simulink model "SingleTrackCANoe"  (R2021b)
settings: Solver=ode1  StartTime=0  StopTime=2  FixedStep=1.0000000000000000e-003  RelTol=1e-3
InitFcn:
  | sampleTime = str2double(get_param(bdroot, 'FixedStep'));
undefined symbols (not defined in the file or in its folder): AccPedalPos, BrakePedalPos, BrakeSwitch, DiscIntNeverNeededParam, DYNA4, EngSpd, IgnitionSwitch, InitialGear, InitialSpeed, IntendedEngTrq, LeftIndicator, MainBrakePress, MaxGear, MDL, MinGear, RefAcc, RefLane, RefLatPos, RefPath, RefPathCurv, RefSpd, RefSpdPreview, RefSpdRetrospect, RightIndicator, SteeringWheelAng, SteeringWheelTrq, UserDefinedRefValue, vm_const
libraries: UtilitiesLibrary x62, simulink x18, WheelSystemModules x14, LongitudinalControllerModules x13, LateralControllerModules x7, AnimationBusselectorModules x5, EnvironmentModules x5, BasicEngineControlModules x5, MiscellaneousControlModules x5, Animation3Modules x4, AuxiliariesModules x4, ReducedTireModules x4
(part 29 of 34)

== system SingleTrackCANoe/SimulationModel/Vehicle/Drivetrain/DrivetrainPhysics/DrivetrainPhysicsOutputs/RearLeftShaftOutput ==
  In1 : Inport
  Bus Selector : BusSelector  OutputSignals=Trq,RotSpd,RotAcc[rad/s**2],DTrqRotAng,DTrqRotSpd,Inrt[kg*m**2],FrictionTrq[Nm]
  RearLeftShaftOutput : Subsystem  Tag=TESIS DYNAware Interface Block  mask{NeedsUpdate=off, SignalInfo=|}
      mask SignalInfo=|
      | {
      |   "Version": "4.6",
      |   "MuxedOutputBusName": "RearLeftShaft",
      |   "MuxedInputBusName": "input",
      |   "MuxedInputSelected": false,
      |   "MuxedOutputSelected": true,
      |   "SignalData": [
      |     {
      |       "initialValue": "0.0",
      |       "name": "Trq[Nm]",
      |       "comment": "",
      |       "minString": "",
      |       "maxString": "",
      |       "width": 1,
      |       "dataType": 0,
      |       "signalType": 0,
      |       "createSignal": false,
      |       "outputName": "Trq[Nm]",
      |       "generateSignalAccessBlock": false,
      |       "accessId": "$(parentId).$(blockName).$(outputName)"
      |     },
      |     {
      |       "initialValue": "0.0",
      |       "name": "RotSpdDifferentialOut[rad/s]",
      |       "comment": "",
      |       "minString": "",
      |       "maxString": "",
      |       "width": 1,
      |       "dataType": 0,
      |       "signalType": 0,
      |       "createSignal": false,
      |       "outputName": "RotSpdDifferentialOut[rad/s]",
      |       "generateSignalAccessBlock": false,
      |       "accessId": "$(parentId).$(blockName).$(outputName)"
      |     },
      |     {
      |       "initialValue": "0.0",
      |       "name": "RotAcc[rad/s**2]",
      |       "comment": "",
      |       "minString": "",
      |       "maxString": "",
      |       "width": 1,
      |       "dataType": 0,
      |       "signalType": 0,
      |       "createSignal": false,
      |       "outputName": "RotAcc[rad/s**2]",
      |       "generateSignalAccessBlock": false,
      |       "accessId": "$(parentId).$(blockName).$(outputName)"
      |     },
      |     {
      |       "initialValue": "0.0",
      |       "name": "DerivativeOfTrq_wrt_RotAng[Nm/rad]",
      |       "comment": "",
      |       "minString": "",
      |       "maxString": "",
      |       "width": 1,
      |       "dataType": 0,
      |       "signalType": 0,
      |       "createSignal": false,
      |       "outputName": "DerivativeOfTrq_wrt_RotAng[Nm/rad]",
      |       "generateSignalAccessBlock": false,
      |       "accessId": "$(parentId).$(blockName).$(outputName)"
      |     },
      |     {
      |       "initialValue": "0.0",
      |       "name": "DerivativeOfTrq_wrt_WheelSpd[Nm/(rad/s)]",
      |       "comment": "",
      |       "minString": "",
      |       "maxString": "",
      |       "width": 1,
      |       "dataType": 0,
      |       "signalType": 0,
      |       "createSignal": false,
      |       "outputName": "DerivativeOfTrq_wrt_WheelSpd[Nm/(rad/s)]",
      |       "generateSignalAccessBlock": false,
      |       "accessId": "$(parentId).$(blockName).$(outputName)"
      |     },
      |     {
      |       "initialValue": "0.0",
      |       "name": "AddInrt[kg*m**2]",
      |       "comment": "",
      |       "minString": "",
      |       "maxString": "",
      |       "width": 1,
      |       "dataType": 0,
      |       "signalType": 0,
      |       "createSignal": false,
      |       "outputName": "AddInrt[kg*m**2]",
      |       "generateSignalAccessBlock": false,
      |       "accessId": "$(parentId).$(blockName).$(outputName)"
      |     },
      |     {
      |       "initialValue": "0.0",
      |       "name": "FrictionTrq[Nm]",
      |       "comment": "",
      |       "minString": "",
      |       "maxString": "",
      |       "width": 1,
      |       "dataType": 0,
      |       "signalType": 0,
      |       "createSignal": false,
      |       "outputName": "FrictionTrq[Nm]",
      |       "generateSignalAccessBlock": false,
      |       "accessId": "$(parentId).$(blockName).$(outputName)"
      |     }
      |   ]
      | }
      mask prompts: NeedsUpdate "Specify, if subsystem content needs to be updated"; SignalInfo "Signal Info (json)"
      mask help: DYNA4 Interface Block Version 4.6
      mask init:
      | blockName = get_param(gcbh, 'Name');
      | parentId = DYNA4.ModelHandling.AccessID.getFromHierarchy(gcbh);
      | TD.InterfaceBlock.ModelCallbacks.GenerateContent(gcb);
      settings: DeleteFcn=TD.InterfaceBlock.ModelCallbacks.CloseGUI( gcbh );  NameChangeFcn=TD.InterfaceBlock.ModelCallbacks.BlockRenamedHandler(gcbh);  OpenFcn=TD.InterfaceBlock.ModelCallbacks.OpenGUI( gcbh );  CloseFcn=TD.InterfaceBlock.ModelCallbacks.CloseGUI( gcbh );
      mask Display:
      | image('InterfaceBlock.png','center');
      | port_label('input',1, 'Trq[Nm]');
      | port_label('input',2, 'RotSpdDifferentialOut[rad/s]');
      | port_label('input',3, 'RotAcc[rad/s**2]');
      | port_label('input',4, 'DerivativeOfTrq_wrt_RotAng[Nm/rad]');
      | port_label('input',5, 'DerivativeOfTrq_wrt_WheelSpd[Nm/(rad/s)]');
      | port_label('input',6, 'AddInrt[kg*m**2]');
      | port_label('input',7, 'FrictionTrq[Nm]');
      | port_label('output',1, 'RearLeftShaft');
  RearLeftShaft : Outport  VectorParamsAs1DForOutWhenUnconnected=off
  wires:
  RearLeftShaftOutput/1(RearLeftShaft___UNIQUE_1) -> RearLeftShaft/1
  In1/1 -> Bus Selector/1
  Bus Selector/1 -> RearLeftShaftOutput/1(Trq[Nm]___UNIQUE_1)  "<Trq>"
  Bus Selector/7 -> RearLeftShaftOutput/7(FrictionTrq[Nm]___UNIQUE_1)  "<FrictionTrq[Nm]>"
  Bus Selector/6 -> RearLeftShaftOutput/6(AddInrt[kg*m**2]___UNIQUE_1)  "<Inrt[kg*m**2]>"
  Bus Selector/4 -> RearLeftShaftOutput/4(DerivativeOfTrq_wrt_RotAng[Nm/rad]___UNIQUE_1)  "<DTrqRotAng>"
  Bus Selector/5 -> RearLeftShaftOutput/5(DerivativeOfTrq_wrt_WheelSpd[Nm/(rad/s)]___UNIQUE_1)  "<DTrqRotSpd>"
  Bus Selector/3 -> RearLeftShaftOutput/3(RotAcc[rad/s**2]___UNIQUE_1)  "<RotAcc[rad/s**2]>"
  Bus Selector/2 -> RearLeftShaftOutput/2(RotSpdDifferentialOut[rad/s]___UNIQUE_1)  "<RotSpd>"

== system SingleTrackCANoe/SimulationModel/Vehicle/Drivetrain/DrivetrainPhysics/DrivetrainPhysicsOutputs/RearRightShaftOutput ==
  In1 : Inport
  Bus Selector : BusSelector  OutputSignals=Trq,RotSpd,RotAcc[rad/s**2],DTrqRotAng,DTrqRotSpd,Inrt[kg*m**2],FrictionTrq[Nm]
  RearRightShaftOutput : Subsystem  Tag=TESIS DYNAware Interface Block  mask{NeedsUpdate=off, SignalInfo=|}
      mask SignalInfo=|
      | {
      |   "Version": "4.6",
      |   "MuxedOutputBusName": "RearRightShaft",
      |   "MuxedInputBusName": "input",
      |   "MuxedInputSelected": false,
      |   "MuxedOutputSelected": true,
      |   "SignalData": [
      |     {
      |       "initialValue": "0.0",
      |       "name": "Trq[Nm]",
      |       "comment": "",
      |       "minString": "",
      |       "maxString": "",
      |       "width": 1,
      |       "dataType": 0,
      |       "signalType": 0,
      |       "createSignal": false,
      |       "outputName": "Trq[Nm]",
      |       "generateSignalAccessBlock": false,
      |       "accessId": "$(parentId).$(blockName).$(outputName)"
      |     },
      |     {
      |       "initialValue": "0.0",
      |       "name": "RotSpdDifferentialOut[rad/s]",
      |       "comment": "",
      |       "minString": "",
      |       "maxString": "",
      |       "width": 1,
      |       "dataType": 0,
      |       "signalType": 0,
      |       "createSignal": false,
      |       "outputName": "RotSpdDifferentialOut[rad/s]",
      |       "generateSignalAccessBlock": false,
      |       "accessId": "$(parentId).$(blockName).$(outputName)"
      |     },
      |     {
      |       "initialValue": "0.0",
      |       "name": "RotAcc[rad/s**2]",
      |       "comment": "",
      |       "minString": "",
      |       "maxString": "",
      |       "width": 1,
      |       "dataType": 0,
      |       "signalType": 0,
      |       "createSignal": false,
      |       "outputName": "RotAcc[rad/s**2]",
      |       "generateSignalAccessBlock": false,
      |       "accessId": "$(parentId).$(blockName).$(outputName)"
      |     },
      |     {
      |       "initialValue": "0.0",
      |       "name": "DerivativeOfTrq_wrt_RotAng[Nm/rad]",
      |       "comment": "",
      |       "minString": "",
      |       "maxString": "",
      |       "width": 1,
      |       "dataType": 0,
      |       "signalType": 0,
      |       "createSignal": false,
      |       "outputName": "DerivativeOfTrq_wrt_RotAng[Nm/rad]",
      |       "generateSignalAccessBlock": false,
      |       "accessId": "$(parentId).$(blockName).$(outputName)"
      |     },
      |     {
      |       "initialValue": "0.0",
      |       "name": "DerivativeOfTrq_wrt_WheelSpd[Nm/(rad/s)]",
      |       "comment": "",
      |       "minString": "",
      |       "maxString": "",
      |       "width": 1,
      |       "dataType": 0,
      |       "signalType": 0,
      |       "createSignal": false,
      |       "outputName": "DerivativeOfTrq_wrt_WheelSpd[Nm/(rad/s)]",
      |       "generateSignalAccessBlock": false,
      |       "accessId": "$(parentId).$(blockName).$(outputName)"
      |     },
      |     {
      |       "initialValue": "0.0",
      |       "name": "AddInrt[kg*m**2]",
      |       "comment": "",
      |       "minString": "",
      |       "maxString": "",
      |       "width": 1,
      |       "dataType": 0,
      |       "signalType": 0,
      |       "createSignal": false,
      |       "outputName": "AddInrt[kg*m**2]",
      |       "generateSignalAccessBlock": false,
      |       "accessId": "$(parentId).$(blockName).$(outputName)"
      |     },
      |     {
      |       "initialValue": "0.0",
      |       "name": "FrictionTrq[Nm]",
      |       "comment": "",
      |       "minString": "",
      |       "maxString": "",
      |       "width": 1,
      |       "dataType": 0,
      |       "signalType": 0,
      |       "createSignal": false,
      |       "outputName": "FrictionTrq[Nm]",
      |       "generateSignalAccessBlock": false,
      |       "accessId": "$(parentId).$(blockName).$(outputName)"
      |     }
      |   ]
      | }
      mask prompts: NeedsUpdate "Specify, if subsystem content needs to be updated"; SignalInfo "Signal Info (json)"
      mask help: DYNA4 Interface Block Version 4.6
      mask init:
      | blockName = get_param(gcbh, 'Name');
      | parentId = DYNA4.ModelHandling.AccessID.getFromHierarchy(gcbh);
      | TD.InterfaceBlock.ModelCallbacks.GenerateContent(gcb);
      settings: DeleteFcn=TD.InterfaceBlock.ModelCallbacks.CloseGUI( gcbh );  NameChangeFcn=TD.InterfaceBlock.ModelCallbacks.BlockRenamedHandler(gcbh);  OpenFcn=TD.InterfaceBlock.ModelCallbacks.OpenGUI( gcbh );  CloseFcn=TD.InterfaceBlock.ModelCallbacks.CloseGUI( gcbh );
      mask Display:
      | image('InterfaceBlock.png','center');
      | port_label('input',1, 'Trq[Nm]');
      | port_label('input',2, 'RotSpdDifferentialOut[rad/s]');
      | port_label('input',3, 'RotAcc[rad/s**2]');
      | port_label('input',4, 'DerivativeOfTrq_wrt_RotAng[Nm/rad]');
      | port_label('input',5, 'DerivativeOfTrq_wrt_WheelSpd[Nm/(rad/s)]');
      | port_label('input',6, 'AddInrt[kg*m**2]');
      | port_label('input',7, 'FrictionTrq[Nm]');
      | port_label('output',1, 'RearRightShaft');
  RearRightShaft : Outport  VectorParamsAs1DForOutWhenUnconnected=off
  wires:
  RearRightShaftOutput/1(RearRightShaft___UNIQUE_1) -> RearRightShaft/1
  In1/1 -> Bus Selector/1
  Bus Selector/1 -> RearRightShaftOutput/1(Trq[Nm]___UNIQUE_1)  "<Trq>"
  Bus Selector/7 -> RearRightShaftOutput/7(FrictionTrq[Nm]___UNIQUE_1)  "<FrictionTrq[Nm]>"
  Bus Selector/6 -> RearRightShaftOutput/6(AddInrt[kg*m**2]___UNIQUE_1)  "<Inrt[kg*m**2]>"
  Bus Selector/4 -> RearRightShaftOutput/4(DerivativeOfTrq_wrt_RotAng[Nm/rad]___UNIQUE_1)  "<DTrqRotAng>"
  Bus Selector/5 -> RearRightShaftOutput/5(DerivativeOfTrq_wrt_WheelSpd[Nm/(rad/s)]___UNIQUE_1)  "<DTrqRotSpd>"
  Bus Selector/3 -> RearRightShaftOutput/3(RotAcc[rad/s**2]___UNIQUE_1)  "<RotAcc[rad/s**2]>"
  Bus Selector/2 -> RearRightShaftOutput/2(RotSpdDifferentialOut[rad/s]___UNIQUE_1)  "<RotSpd>"

== system SingleTrackCANoe/SimulationModel/Vehicle/Drivetrain/DrivetrainPhysics/DrivetrainPhysicsOutputs/TotalRatio ==
  TransmissionStates : Inport
  OutputDriveRatio : Inport  Port=2
  Bus Selector16 : BusSelector  OutputSignals=Ratio[-]
  Product : Product  RndMeth=Zero
  TotalRatio : Outport  VectorParamsAs1DForOutWhenUnconnected=off
  wires:
  Product/1 -> TotalRatio/1
  OutputDriveRatio/1 -> Product/2
  TransmissionStates/1 -> Bus Selector16/1
  Bus Selector16/1 -> Product/1  "<Ratio[-]>"

== system SingleTrackCANoe/SimulationModel/Vehicle/Drivetrain/DrivetrainPhysics/DrivetrainPhysicsOutputs/TransferCaseOutput ==
  TransferCaseStates : Inport
  Bus Selector : BusSelector  OutputSignals=TrqDistributionFac[0_1]
  TransferCaseOutput : Subsystem  Tag=TESIS DYNAware Interface Block  mask{NeedsUpdate=off, SignalInfo=|}
      mask SignalInfo=|
      | {
      |   "Version": "4.6",
      |   "MuxedOutputBusName": "TransferCase",
      |   "MuxedInputBusName": "input",
      |   "MuxedInputSelected": false,
      |   "MuxedOutputSelected": true,
      |   "SignalData": {
      |     "initialValue": "0.0",
      |     "name": "TrqDistributionFac[0_1]",
      |     "comment": "",
      |     "minString": "",
      |     "maxString": "",
      |     "width": 1,
      |     "dataType": 0,
      |     "signalType": 0,
      |     "createSignal": false,
      |     "outputName": "TrqDistributionFac[0_1]",
      |     "generateSignalAccessBlock": false,
      |     "accessId": "$(parentId).$(blockName).$(outputName)"
      |   }
      | }
      mask prompts: NeedsUpdate "Specify, if subsystem content needs to be updated"; SignalInfo "Signal Info (json)"
      mask help: DYNA4 Interface Block Version 4.6
      mask init:
      | blockName = get_param(gcbh, 'Name');
      | parentId = DYNA4.ModelHandling.AccessID.getFromHierarchy(gcbh);
      | TD.InterfaceBlock.ModelCallbacks.GenerateContent(gcb);
      settings: DeleteFcn=TD.InterfaceBlock.ModelCallbacks.CloseGUI( gcbh );  NameChangeFcn=TD.InterfaceBlock.ModelCallbacks.BlockRenamedHandler(gcbh);  OpenFcn=TD.InterfaceBlock.ModelCallbacks.OpenGUI( gcbh );  CloseFcn=TD.InterfaceBlock.ModelCallbacks.CloseGUI( gcbh );
      mask Display:
      | image('InterfaceBlock.png','center');
      | port_label('input',1, 'TrqDistributionFac[0_1]');
      | port_label('output',1, 'TransferCase');
  TransferCase : Outport  VectorParamsAs1DForOutWhenUnconnected=off
  wires:
  TransferCaseStates/1 -> Bus Selector/1
  TransferCaseOutput/1(TransferCase___UNIQUE_1) -> TransferCase/1
  Bus Selector/1 -> TransferCaseOutput/1(TrqDistributionFac[0_1]___UNIQUE_1)  "<TrqDistributionFac[0_1]>"

== system SingleTrackCANoe/SimulationModel/Vehicle/Drivetrain/DrivetrainPhysics/DrivetrainPhysicsOutputs/TransmissionOutput ==
  TransmissionStates : Inport
  Bus Selector : BusSelector  OutputSignals=NumFwdGears,Type[-],Gear[-4;20],InSpd[rad/s],OutSpd[rad/s],GearChangeTimeConst
  TransmissionOutput : Subsystem  Tag=TESIS DYNAware Interface Block  mask{NeedsUpdate=off, SignalInfo=|}
      mask SignalInfo=|
      | {
      |   "Version": "4.6",
      |   "MuxedOutputBusName": "Transmission",
      |   "MuxedInputBusName": "input",
      |   "MuxedInputSelected": false,
      |   "MuxedOutputSelected": true,
      |   "SignalData": [
      |     {
      |       "initialValue": "0.0",
      |       "name": "NumFwdGears[-]",
      |       "comment": "",
      |       "minString": "",
      |       "maxString": "",
      |       "width": 1,
      |       "dataType": 0,
      |       "signalType": 0,
      |       "createSignal": false,
      |       "outputName": "NumFwdGears[-]",
      |       "generateSignalAccessBlock": false,
      |       "accessId": "$(parentId).$(blockName).$(outputName)"
      |     },
      |     {
      |       "initialValue": "0.0",
      |       "name": "Type[-]",
      |       "comment": "",
      |       "minString": "",
      |       "maxString": "",
      |       "width": 1,
      |       "dataType": 0,
      |       "signalType": 0,
      |       "createSignal": false,
      |       "outputName": "Type[-]",
      |       "generateSignalAccessBlock": false,
      |       "accessId": "$(parentId).$(blockName).$(outputName)"
      |     },
      |     {
      |       "initialValue": "0.0",
      |       "name": "Gear[-4;20]",
      |       "comment": "",
      |       "minString": "",
      |       "maxString": "",
      |       "width": 1,
      |       "dataType": 0,
      |       "signalType": 0,
      |       "createSignal": false,
      |       "outputName": "Gear[-4;20]",
      |       "generateSignalAccessBlock": false,
      |       "accessId": "$(parentId).$(blockName).$(outputName)"
      |     },
      |     {
      |       "initialValue": "0.0",
      |       "name": "InSpd[rad/s]",
      |       "comment": "",
      |       "minString": "",
      |       "maxString": "",
      |       "width": 1,
      |       "dataType": 0,
      |       "signalType": 0,
      |       "createSignal": false,
      |       "outputName": "InSpd[rad/s]",
      |       "generateSignalAccessBlock": false,
      |       "accessId": "$(parentId).$(blockName).$(outputName)"
      |     },
      |     {
      |       "initialValue": "0.0",
      |       "name": "OutSpd[rad/s]",
      |       "comment": "",
      |       "minString": "",
      |       "maxString": "",
      |       "width": 1,
      |       "dataType": 0,
      |       "signalType": 0,
      |       "createSignal": false,
      |       "outputName": "OutSpd[rad/s]",
      |       "generateSignalAccessBlock": false,
      |       "accessId": "$(parentId).$(blockName).$(outputName)"
      |     },
      |     {
      |       "initialValue": "0.0",
      |       "name": "GearChangeTimeConst[s]",
      |       "comment": "",
      |       "minString": "",
      |       "maxString": "",
      |       "width": 1,
      |       "dataType": 0,
      |       "signalType": 0,
      |       "createSignal": false,
      |       "outputName": "GearChangeTimeConst[s]",
      |       "generateSignalAccessBlock": false,
      |       "accessId": "$(parentId).$(blockName).$(outputName)"
      |     }
      |   ]
      | }
      mask prompts: NeedsUpdate "Specify, if subsystem content needs to be updated"; SignalInfo "Signal Info (json)"
      mask help: DYNA4 Interface Block Version 4.6
      mask init:
      | blockName = get_param(gcbh, 'Name');
      | parentId = DYNA4.ModelHandling.AccessID.getFromHierarchy(gcbh);
      | TD.InterfaceBlock.ModelCallbacks.GenerateContent(gcb);
      settings: DeleteFcn=TD.InterfaceBlock.ModelCallbacks.CloseGUI( gcbh );  NameChangeFcn=TD.InterfaceBlock.ModelCallbacks.BlockRenamedHandler(gcbh);  OpenFcn=TD.InterfaceBlock.ModelCallbacks.OpenGUI( gcbh );  CloseFcn=TD.InterfaceBlock.ModelCallbacks.CloseGUI( gcbh );
      mask Display:
      | image('InterfaceBlock.png','center');
      | port_label('input',1, 'NumFwdGears[-]');
      | port_label('input',2, 'Type[-]');
      | port_label('input',3, 'Gear[-4;20]');
      | port_label('input',4, 'InSpd[rad/s]');
      | port_label('input',5, 'OutSpd[rad/s]');
      | port_label('input',6, 'GearChangeTimeConst[s]');
      | port_label('output',1, 'Transmission');
  Transmission : Outport  VectorParamsAs1DForOutWhenUnconnected=off
  wires:
  TransmissionOutput/1(Transmission___UNIQUE_1) -> Transmission/1
  TransmissionStates/1 -> Bus Selector/1
  Bus Selector/2 -> TransmissionOutput/2(Type[-]___UNIQUE_1)  "<Type[-]>"
  Bus Selector/1 -> TransmissionOutput/1(NumFwdGears[-]___UNIQUE_1)  "<NumFwdGears>"
  Bus Selector/6 -> TransmissionOutput/6(GearChangeTimeConst[s]___UNIQUE_1)  "<GearChangeTimeConst>"
  Bus Selector/3 -> TransmissionOutput/3(Gear[-4;20]___UNIQUE_1)  "<Gear[-4;20]>"
  Bus Selector/4 -> TransmissionOutput/4(InSpd[rad/s]___UNIQUE_1)  "<InSpd[rad/s]>"
  Bus Selector/5 -> TransmissionOutput/5(OutSpd[rad/s]___UNIQUE_1)  "<OutSpd[rad/s]>"

== system SingleTrackCANoe/SimulationModel/Vehicle/WheelSystem/FrontLeftWheelSystem/Tire/DynaComponentInfo ==

== system SingleTrackCANoe/SimulationModel/Vehicle/WheelSystem/FrontLeftWheelSystem/Tire/InputFromCTRL ==
  fromCTRL : Inport
  TDBusSelector : BusSelector  OutputSignals=AddRoadElev[m],RoadFrictionScaling[0_2],AddLongRoadSlope[-],AddLatRoadSlope[-],LocalRoadSysSwitch[0;1]
  __TDD__AddLatRoadSlope[-] : Demux  Outputs=[1]
  __TDD__AddLongRoadSlope[-] : Demux  Outputs=[1]
  __TDD__AddRoadElev[m] : Demux  Outputs=[1]
  __TDD__LocalRoadSysSwitch[0;1] : Demux  Outputs=[1]
  __TDD__RoadFrictionScaling[0_2] : Demux  Outputs=[1]
  AddRoadElev[m]___UNIQUE_1 : Outport  Description=|  PortDimensions=[1]  VectorParamsAs1DForOutWhenUnconnected=off
      | <name>AddRoadElev[m]</name>
      | <comment></comment>
  RoadFrictionScaling[0_2]___UNIQUE_1 : Outport  Description=|  Port=2  PortDimensions=[1]  VectorParamsAs1DForOutWhenUnconnected=off
      | <name>RoadFrictionScaling[0_2]</name>
      | <comment></comment>
  AddLongRoadSlope[-]___UNIQUE_1 : Outport  Description=|  Port=3  PortDimensions=[1]  VectorParamsAs1DForOutWhenUnconnected=off
      | <name>AddLongRoadSlope[-]</name>
      | <comment></comment>
  AddLatRoadSlope[-]___UNIQUE_1 : Outport  Description=|  Port=4  PortDimensions=[1]  VectorParamsAs1DForOutWhenUnconnected=off
      | <name>AddLatRoadSlope[-]</name>
      | <comment></comment>
  LocalRoadSysSwitch[0;1]___UNIQUE_1 : Outport  Description=|  Port=5  PortDimensions=[1]  VectorParamsAs1DForOutWhenUnconnected=off
      | <name>LocalRoadSysSwitch[0;1]</name>
      | <comment></comment>
  wires:
  fromCTRL/1 -> TDBusSelector/1
  TDBusSelector/1 -> __TDD__AddRoadElev[m]/1  "<AddRoadElev[m]>"
  TDBusSelector/2 -> __TDD__RoadFrictionScaling[0_2]/1  "<RoadFrictionScaling[0_2]>"
  TDBusSelector/3 -> __TDD__AddLongRoadSlope[-]/1  "<AddLongRoadSlope[-]>"
  TDBusSelector/4 -> __TDD__AddLatRoadSlope[-]/1  "<AddLatRoadSlope[-]>"
  TDBusSelector/5 -> __TDD__LocalRoadSysSwitch[0;1]/1  "<LocalRoadSysSwitch[0;1]>"
  __TDD__AddRoadElev[m]/1 -> AddRoadElev[m]___UNIQUE_1/1  "AddRoadElev[m]"
  __TDD__RoadFrictionScaling[0_2]/1 -> RoadFrictionScaling[0_2]___UNIQUE_1/1  "RoadFrictionScaling[0_2]"
  __TDD__AddLongRoadSlope[-]/1 -> AddLongRoadSlope[-]___UNIQUE_1/1  "AddLongRoadSlope[-]"
  __TDD__AddLatRoadSlope[-]/1 -> AddLatRoadSlope[-]___UNIQUE_1/1  "AddLatRoadSlope[-]"
  __TDD__LocalRoadSysSwitch[0;1]/1 -> LocalRoadSysSwitch[0;1]___UNIQUE_1/1  "LocalRoadSysSwitch[0;1]"

== system SingleTrackCANoe/SimulationModel/Vehicle/WheelSystem/FrontLeftWheelSystem/Tire/InputFromChassis ==
  fromChassis : Inport
  TDBusSelector : BusSelector  OutputSignals=VehicleBody.PosAxleSys(WorldSys),VehicleBody.RotMatrix(WorldSys)[-],WheelSystem.WheelRotAxis(VehSys)[-],WheelSystem.TirePos(AxleSys)[m],WheelSystem.TireVel_wrt_WorldSys(VehSys)[m/s],WheelSystem.WheelRotVel_wrt_WorldSys(VehSys)[rad/s],VehicleBody.Vel_wrt_WorldSys(VehSys)[m/s],WheelSystem.WheelRotMatrix(WorldSys)[-],WheelSystem.TireDefl[m]
  __TDD__PosAxleSys(WorldSys) : Demux  Outputs=1
  __TDD__RotMatrix(WorldSys)[-] : Demux  Outputs=[9]
  __TDD__TireDefl[m] : Demux  Outputs=[1]
  __TDD__TirePos(AxleSys)[m] : Demux  Outputs=1
  __TDD__TireVel_wrt_WorldSys(VehSys)[m/s] : Demux  Outputs=[3]
  __TDD__Vel_wrt_WorldSys(VehSys)[m/s] : Demux  Outputs=[3]
  __TDD__WheelRotAxis(VehSys)[-] : Demux  Outputs=[3]
  __TDD__WheelRotMatrix(WorldSys)[-] : Demux  Outputs=[9]
  __TDD__WheelRotVel_wrt_WorldSys(VehSys)[rad/s] : Demux  Outputs=[3]
  PosAxleSys(WorldSys)___UNIQUE_1 : Outport  Description=|  VectorParamsAs1DForOutWhenUnconnected=off
      | <name>VehicleBody.PosAxleSys(WorldSys)</name>
      | <comment></comment>
  RotMatrix(WorldSys)[-]___UNIQUE_1 : Outport  Description=|  Port=2  PortDimensions=[9]  VectorParamsAs1DForOutWhenUnconnected=off
      | <name>VehicleBody.RotMatrix(WorldSys)[-]</name>
      | <comment></comment>
  WheelRotAxis(VehSys)[-]___UNIQUE_1 : Outport  Description=|  Port=3  PortDimensions=[3]  VectorParamsAs1DForOutWhenUnconnected=off
      | <name>WheelSystem.WheelRotAxis(VehSys)[-]</name>
      | <comment></comment>
  TirePos(AxleSys)[m]___UNIQUE_1 : Outport  Description=|  Port=4  VectorParamsAs1DForOutWhenUnconnected=off
      | <name>WheelSystem.TirePos(AxleSys)[m]</name>
      | <comment></comment>
  TireVel_wrt_WorldSys(VehSys)[m/s]___UNIQUE_1 : Outport  Description=|  Port=5  PortDimensions=[3]  VectorParamsAs1DForOutWhenUnconnected=off
      | <name>WheelSystem.TireVel_wrt_WorldSys(VehSys)[m/s]</name>
      | <comment></comment>
  WheelRotVel_wrt_WorldSys(VehSys)[rad/s]___UNIQUE_1 : Outport  Description=|  Port=6  PortDimensions=[3]  VectorParamsAs1DForOutWhenUnconnected=off
      | <name>WheelSystem.WheelRotVel_wrt_WorldSys(VehSys)[rad/s]</name>
      | <comment></comment>
  Vel_wrt_WorldSys(VehSys)[m/s]___UNIQUE_1 : Outport  Description=|  Port=7  PortDimensions=[3]  VectorParamsAs1DForOutWhenUnconnected=off
      | <name>VehicleBody.Vel_wrt_WorldSys(VehSys)[m/s]</name>
      | <comment></comment>
  WheelRotMatrix(WorldSys)[-]___UNIQUE_1 : Outport  Description=|  Port=8  PortDimensions=[9]  VectorParamsAs1DForOutWhenUnconnected=off
      | <name>WheelSystem.WheelRotMatrix(WorldSys)[-]</name>
      | <comment></comment>
  TireDefl[m]___UNIQUE_1 : Outport  Description=|  Port=9  PortDimensions=[1]  VectorParamsAs1DForOutWhenUnconnected=off
      | <name>WheelSystem.TireDefl[m]</name>
      | <comment></comment>
  wires:
  fromChassis/1 -> TDBusSelector/1
  TDBusSelector/1 -> __TDD__PosAxleSys(WorldSys)/1  "<PosAxleSys(WorldSys)>"
  TDBusSelector/2 -> __TDD__RotMatrix(WorldSys)[-]/1  "<RotMatrix(WorldSys)[-]>"
  TDBusSelector/3 -> __TDD__WheelRotAxis(VehSys)[-]/1  "<WheelRotAxis(VehSys)[-]>"
  TDBusSelector/4 -> __TDD__TirePos(AxleSys)[m]/1  "<TirePos(AxleSys)[m]>"
  TDBusSelector/5 -> __TDD__TireVel_wrt_WorldSys(VehSys)[m/s]/1  "<TireVel_wrt_WorldSys(VehSys)[m/s]>"
  TDBusSelector/6 -> __TDD__WheelRotVel_wrt_WorldSys(VehSys)[rad/s]/1  "<WheelRotVel_wrt_WorldSys(VehSys)[rad/s]>"
  TDBusSelector/7 -> __TDD__Vel_wrt_WorldSys(VehSys)[m/s]/1  "<Vel_wrt_WorldSys(VehSys)[m/s]>"
  TDBusSelector/8 -> __TDD__WheelRotMatrix(WorldSys)[-]/1  "<WheelRotMatrix(WorldSys)[-]>"
  TDBusSelector/9 -> __TDD__TireDefl[m]/1  "<TireDefl[m]>"
  __TDD__PosAxleSys(WorldSys)/1 -> PosAxleSys(WorldSys)___UNIQUE_1/1  "PosAxleSys(WorldSys)"
  __TDD__RotMatrix(WorldSys)[-]/1 -> RotMatrix(WorldSys)[-]___UNIQUE_1/1  "RotMatrix(WorldSys)[-]"
  __TDD__WheelRotAxis(VehSys)[-]/1 -> WheelRotAxis(VehSys)[-]___UNIQUE_1/1  "WheelRotAxis(VehSys)[-]"
  __TDD__TirePos(AxleSys)[m]/1 -> TirePos(AxleSys)[m]___UNIQUE_1/1  "TirePos(AxleSys)[m]"
  __TDD__TireVel_wrt_WorldSys(VehSys)[m/s]/1 -> TireVel_wrt_WorldSys(VehSys)[m/s]___UNIQUE_1/1  "TireVel_wrt_WorldSys(VehSys)[m/s]"
  __TDD__WheelRotVel_wrt_WorldSys(VehSys)[rad/s]/1 -> WheelRotVel_wrt_WorldSys(VehSys)[rad/s]___UNIQUE_1/1  "WheelRotVel_wrt_WorldSys(VehSys)[rad/s]"
  __TDD__Vel_wrt_WorldSys(VehSys)[m/s]/1 -> Vel_wrt_WorldSys(VehSys)[m/s]___UNIQUE_1/1  "Vel_wrt_WorldSys(VehSys)[m/s]"
  __TDD__WheelRotMatrix(WorldSys)[-]/1 -> WheelRotMatrix(WorldSys)[-]___UNIQUE_1/1  "WheelRotMatrix(WorldSys)[-]"
  __TDD__TireDefl[m]/1 -> TireDefl[m]___UNIQUE_1/1  "TireDefl[m]"

== system SingleTrackCANoe/SimulationModel/Vehicle/WheelSystem/FrontLeftWheelSystem/Tire/InputFromWheel ==
  fromWheel : Inport
  TDBusSelector : BusSelector  OutputSignals=RotSpd[rad/s],BlockingState[0;1]
  __TDD__BlockingState[0;1] : Demux  Outputs=[1]
  __TDD__RotSpd[rad/s] : Demux  Outputs=[1]
  RotSpd[rad/s]___UNIQUE_1 : Outport  Description=|  PortDimensions=[1]  VectorParamsAs1DForOutWhenUnconnected=off
      | <name>RotSpd[rad/s]</name>
      | <comment></comment>
  BlockingState[0;1]___UNIQUE_1 : Outport  Description=|  Port=2  PortDimensions=[1]  VectorParamsAs1DForOutWhenUnconnected=off
      | <name>BlockingState[0;1]</name>
      | <comment></comment>
  wires:
  fromWheel/1 -> TDBusSelector/1
  TDBusSelector/1 -> __TDD__RotSpd[rad/s]/1  "<RotSpd[rad/s]>"
  TDBusSelector/2 -> __TDD__BlockingState[0;1]/1  "<BlockingState[0;1]>"
  __TDD__RotSpd[rad/s]/1 -> RotSpd[rad/s]___UNIQUE_1/1  "RotSpd[rad/s]"
  __TDD__BlockingState[0;1]/1 -> BlockingState[0;1]___UNIQUE_1/1  "BlockingState[0;1]"

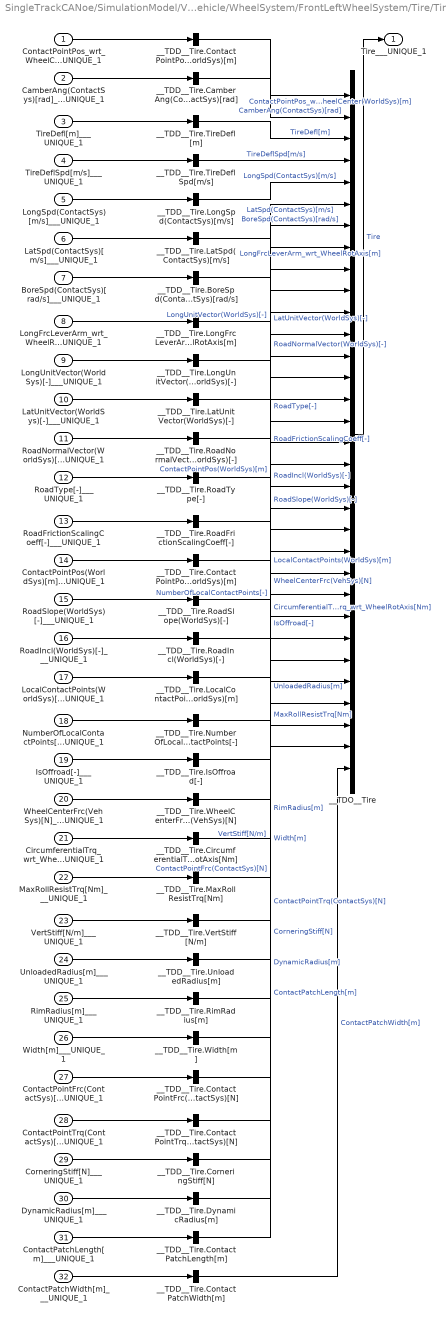
== system SingleTrackCANoe/SimulationModel/Vehicle/WheelSystem/FrontLeftWheelSystem/Tire/Tire Output ==
  ContactPointPos_wrt_WheelCenter(WorldSys)[m]___UNIQUE_1 : Inport  Description=|  PortDimensions=[3]
      | <name>ContactPointPos_wrt_WheelCenter(WorldSys)[m]</name>
      | <comment></comment>
  CamberAng(ContactSys)[rad]___UNIQUE_1 : Inport  Description=|  Port=2  PortDimensions=[1]
      | <name>CamberAng(ContactSys)[rad]</name>
      | <comment></comment>
  TireDefl[m]___UNIQUE_1 : Inport  Description=|  Port=3  PortDimensions=[1]
      | <name>TireDefl[m]</name>
      | <comment></comment>
  TireDeflSpd[m/s]___UNIQUE_1 : Inport  Description=|  Port=4  PortDimensions=[1]
      | <name>TireDeflSpd[m/s]</name>
      | <comment></comment>
  LongSpd(ContactSys)[m/s]___UNIQUE_1 : Inport  Description=|  Port=5  PortDimensions=[1]
      | <name>LongSpd(ContactSys)[m/s]</name>
      | <comment></comment>
  LatSpd(ContactSys)[m/s]___UNIQUE_1 : Inport  Description=|  Port=6  PortDimensions=[1]
      | <name>LatSpd(ContactSys)[m/s]</name>
      | <comment></comment>
  BoreSpd(ContactSys)[rad/s]___UNIQUE_1 : Inport  Description=|  Port=7  PortDimensions=[1]
      | <name>BoreSpd(ContactSys)[rad/s]</name>
      | <comment></comment>
  LongFrcLeverArm_wrt_WheelRotAxis[m]___UNIQUE_1 : Inport  Description=|  Port=8  PortDimensions=[1]
      | <name>LongFrcLeverArm_wrt_WheelRotAxis[m]</name>
      | <comment></comment>
  LongUnitVector(WorldSys)[-]___UNIQUE_1 : Inport  Description=|  Port=9  PortDimensions=[3]
      | <name>LongUnitVector(WorldSys)[-]</name>
      | <comment></comment>
  LatUnitVector(WorldSys)[-]___UNIQUE_1 : Inport  Description=|  Port=10  PortDimensions=[3]
      | <name>LatUnitVector(WorldSys)[-]</name>
      | <comment></comment>
  RoadNormalVector(WorldSys)[-]___UNIQUE_1 : Inport  Description=|  Port=11  PortDimensions=[3]
      | <name>RoadNormalVector(WorldSys)[-]</name>
      | <comment></comment>
  RoadType[-]___UNIQUE_1 : Inport  Description=|  Port=12  PortDimensions=[1]
      | <name>RoadType[-]</name>
      | <comment></comment>
  RoadFrictionScalingCoeff[-]___UNIQUE_1 : Inport  Description=|  Port=13  PortDimensions=[1]
      | <name>RoadFrictionScalingCoeff[-]</name>
      | <comment></comment>
  ContactPointPos(WorldSys)[m]___UNIQUE_1 : Inport  Description=|  Port=14  PortDimensions=[3]
      | <name>ContactPointPos(WorldSys)[m]</name>
      | <comment></comment>
  RoadSlope(WorldSys)[-]___UNIQUE_1 : Inport  Description=|  Port=15  PortDimensions=[1]
      | <name>RoadSlope(WorldSys)[-]</name>
      | <comment></comment>
  RoadIncl(WorldSys)[-]___UNIQUE_1 : Inport  Description=|  Port=16  PortDimensions=[1]
      | <name>RoadIncl(WorldSys)[-]</name>
      | <comment></comment>
  LocalContactPoints(WorldSys)[m]___UNIQUE_1 : Inport  Description=|  Port=17  PortDimensions=[12]
      | <name>LocalContactPoints(WorldSys)[m]</name>
      | <comment></comment>
  NumberOfLocalContactPoints[-]___UNIQUE_1 : Inport  Description=|  Port=18  PortDimensions=[1]
      | <name>NumberOfLocalContactPoints[-]</name>
      | <comment></comment>
  IsOffroad[-]___UNIQUE_1 : Inport  Description=|  Port=19  PortDimensions=[1]
      | <name>IsOffroad[-]</name>
      | <comment></comment>
  WheelCenterFrc(VehSys)[N]___UNIQUE_1 : Inport  Description=|  Port=20  PortDimensions=[3]
      | <name>WheelCenterFrc(VehSys)[N]</name>
      | <comment></comment>
  CircumferentialTrq_wrt_WheelRotAxis[Nm]___UNIQUE_1 : Inport  Description=|  Port=21  PortDimensions=[1]
      | <name>CircumferentialTrq_wrt_WheelRotAxis[Nm]</name>
      | <comment></comment>
  MaxRollResistTrq[Nm]___UNIQUE_1 : Inport  Description=|  Port=22  PortDimensions=[1]
      | <name>MaxRollResistTrq[Nm]</name>
      | <comment></comment>
  VertStiff[N/m]___UNIQUE_1 : Inport  Description=|  Port=23  PortDimensions=[1]
      | <name>VertStiff[N/m]</name>
      | <comment></comment>
  UnloadedRadius[m]___UNIQUE_1 : Inport  Description=|  Port=24  PortDimensions=[1]
      | <name>UnloadedRadius[m]</name>
      | <comment></comment>
  RimRadius[m]___UNIQUE_1 : Inport  Description=|  Port=25  PortDimensions=[1]
      | <name>RimRadius[m]</name>
      | <comment></comment>
  Width[m]___UNIQUE_1 : Inport  Description=|  Port=26  PortDimensions=[1]
      | <name>Width[m]</name>
      | <comment></comment>
  ContactPointFrc(ContactSys)[N]___UNIQUE_1 : Inport  Description=|  Port=27  PortDimensions=[3]
      | <name>ContactPointFrc(ContactSys)[N]</name>
      | <comment></comment>
  ContactPointTrq(ContactSys)[N]___UNIQUE_1 : Inport  Description=|  Port=28  PortDimensions=[3]
      | <name>ContactPointTrq(ContactSys)[N]</name>
      | <comment></comment>
  CorneringStiff[N]___UNIQUE_1 : Inport  Description=|  Port=29  PortDimensions=[1]
      | <name>CorneringStiff[N]</name>
      | <comment></comment>
  DynamicRadius[m]___UNIQUE_1 : Inport  Description=|  Port=30  PortDimensions=[1]
      | <name>DynamicRadius[m]</name>
      | <comment></comment>
  ContactPatchLength[m]___UNIQUE_1 : Inport  Description=|  Port=31  PortDimensions=[1]
      | <name>ContactPatchLength[m]</name>
      | <comment></comment>
  ContactPatchWidth[m]___UNIQUE_1 : Inport  Description=|  Port=32  PortDimensions=[1]
      | <name>ContactPatchWidth[m]</name>
      | <comment></comment>
  __TDD__Tire.BoreSpd(ContactSys)[rad/s] : Demux  Outputs=[1]
  __TDD__Tire.CamberAng(ContactSys)[rad] : Demux  Outputs=[1]
  __TDD__Tire.CircumferentialTrq_wrt_WheelRotAxis[Nm] : Demux  Outputs=[1]
  __TDD__Tire.ContactPatchLength[m] : Demux  Outputs=[1]
  __TDD__Tire.ContactPatchWidth[m] : Demux  Outputs=[1]
  __TDD__Tire.ContactPointFrc(ContactSys)[N] : Demux  Outputs=[3]
  __TDD__Tire.ContactPointPos(WorldSys)[m] : Demux  Outputs=[3]
  __TDD__Tire.ContactPointPos_wrt_WheelCenter(WorldSys)[m] : Demux  Outputs=[3]
  __TDD__Tire.ContactPointTrq(ContactSys)[N] : Demux  Outputs=[3]
  __TDD__Tire.CorneringStiff[N] : Demux  Outputs=[1]
  __TDD__Tire.DynamicRadius[m] : Demux  Outputs=[1]
  __TDD__Tire.IsOffroad[-] : Demux  Outputs=[1]
  __TDD__Tire.LatSpd(ContactSys)[m/s] : Demux  Outputs=[1]
  __TDD__Tire.LatUnitVector(WorldSys)[-] : Demux  Outputs=[3]
  __TDD__Tire.LocalContactPoints(WorldSys)[m] : Demux  Outputs=[12]
  __TDD__Tire.LongFrcLeverArm_wrt_WheelRotAxis[m] : Demux  Outputs=[1]
  __TDD__Tire.LongSpd(ContactSys)[m/s] : Demux  Outputs=[1]
  __TDD__Tire.LongUnitVector(WorldSys)[-] : Demux  Outputs=[3]
  __TDD__Tire.MaxRollResistTrq[Nm] : Demux  Outputs=[1]
  __TDD__Tire.NumberOfLocalContactPoints[-] : Demux  Outputs=[1]
  __TDD__Tire.RimRadius[m] : Demux  Outputs=[1]
  __TDD__Tire.RoadFrictionScalingCoeff[-] : Demux  Outputs=[1]
  __TDD__Tire.RoadIncl(WorldSys)[-] : Demux  Outputs=[1]
  __TDD__Tire.RoadNormalVector(WorldSys)[-] : Demux  Outputs=[3]
  __TDD__Tire.RoadSlope(WorldSys)[-] : Demux  Outputs=[1]
  __TDD__Tire.RoadType[-] : Demux  Outputs=[1]
  __TDD__Tire.TireDeflSpd[m/s] : Demux  Outputs=[1]
  __TDD__Tire.TireDefl[m] : Demux  Outputs=[1]
  __TDD__Tire.UnloadedRadius[m] : Demux  Outputs=[1]
  __TDD__Tire.VertStiff[N/m] : Demux  Outputs=[1]
  __TDD__Tire.WheelCenterFrc(VehSys)[N] : Demux  Outputs=[3]
  __TDD__Tire.Width[m] : Demux  Outputs=[1]
  __TDO__Tire : BusCreator  Inputs=32
  Tire___UNIQUE_1 : Outport  Description=|  PortDimensions=[59]  VectorParamsAs1DForOutWhenUnconnected=off
      | <name>ContactPointPos_wrt_WheelCenter(WorldSys)[m]</name>
      | <comment></comment>
  wires:
  __TDO__Tire/1 -> Tire___UNIQUE_1/1  "Tire"
  __TDD__Tire.ContactPatchWidth[m]/1 -> __TDO__Tire/32  "ContactPatchWidth[m]"
  ContactPatchWidth[m]___UNIQUE_1/1 -> __TDD__Tire.ContactPatchWidth[m]/1
  __TDD__Tire.ContactPatchLength[m]/1 -> __TDO__Tire/31  "ContactPatchLength[m]"
  ContactPatchLength[m]___UNIQUE_1/1 -> __TDD__Tire.ContactPatchLength[m]/1
  __TDD__Tire.DynamicRadius[m]/1 -> __TDO__Tire/30  "DynamicRadius[m]"
  DynamicRadius[m]___UNIQUE_1/1 -> __TDD__Tire.DynamicRadius[m]/1
  __TDD__Tire.CorneringStiff[N]/1 -> __TDO__Tire/29  "CorneringStiff[N]"
  CorneringStiff[N]___UNIQUE_1/1 -> __TDD__Tire.CorneringStiff[N]/1
  __TDD__Tire.ContactPointTrq(ContactSys)[N]/1 -> __TDO__Tire/28  "ContactPointTrq(ContactSys)[N]"
  ContactPointTrq(ContactSys)[N]___UNIQUE_1/1 -> __TDD__Tire.ContactPointTrq(ContactSys)[N]/1
  __TDD__Tire.ContactPointFrc(ContactSys)[N]/1 -> __TDO__Tire/27  "ContactPointFrc(ContactSys)[N]"
  ContactPointFrc(ContactSys)[N]___UNIQUE_1/1 -> __TDD__Tire.ContactPointFrc(ContactSys)[N]/1
  __TDD__Tire.Width[m]/1 -> __TDO__Tire/26  "Width[m]"
  Width[m]___UNIQUE_1/1 -> __TDD__Tire.Width[m]/1
  __TDD__Tire.RimRadius[m]/1 -> __TDO__Tire/25  "RimRadius[m]"
  RimRadius[m]___UNIQUE_1/1 -> __TDD__Tire.RimRadius[m]/1
  __TDD__Tire.UnloadedRadius[m]/1 -> __TDO__Tire/24  "UnloadedRadius[m]"
  UnloadedRadius[m]___UNIQUE_1/1 -> __TDD__Tire.UnloadedRadius[m]/1
  __TDD__Tire.VertStiff[N/m]/1 -> __TDO__Tire/23  "VertStiff[N/m]"
  VertStiff[N/m]___UNIQUE_1/1 -> __TDD__Tire.VertStiff[N/m]/1
  __TDD__Tire.MaxRollResistTrq[Nm]/1 -> __TDO__Tire/22  "MaxRollResistTrq[Nm]"
  MaxRollResistTrq[Nm]___UNIQUE_1/1 -> __TDD__Tire.MaxRollResistTrq[Nm]/1
  __TDD__Tire.CircumferentialTrq_wrt_WheelRotAxis[Nm]/1 -> __TDO__Tire/21  "CircumferentialTrq_wrt_WheelRotAxis[Nm]"
  CircumferentialTrq_wrt_WheelRotAxis[Nm]___UNIQUE_1/1 -> __TDD__Tire.CircumferentialTrq_wrt_WheelRotAxis[Nm]/1
  __TDD__Tire.WheelCenterFrc(VehSys)[N]/1 -> __TDO__Tire/20  "WheelCenterFrc(VehSys)[N]"
  WheelCenterFrc(VehSys)[N]___UNIQUE_1/1 -> __TDD__Tire.WheelCenterFrc(VehSys)[N]/1
  __TDD__Tire.IsOffroad[-]/1 -> __TDO__Tire/19  "IsOffroad[-]"
  IsOffroad[-]___UNIQUE_1/1 -> __TDD__Tire.IsOffroad[-]/1
  __TDD__Tire.NumberOfLocalContactPoints[-]/1 -> __TDO__Tire/18  "NumberOfLocalContactPoints[-]"
  NumberOfLocalContactPoints[-]___UNIQUE_1/1 -> __TDD__Tire.NumberOfLocalContactPoints[-]/1
  __TDD__Tire.LocalContactPoints(WorldSys)[m]/1 -> __TDO__Tire/17  "LocalContactPoints(WorldSys)[m]"
  LocalContactPoints(WorldSys)[m]___UNIQUE_1/1 -> __TDD__Tire.LocalContactPoints(WorldSys)[m]/1
  __TDD__Tire.RoadIncl(WorldSys)[-]/1 -> __TDO__Tire/16  "RoadIncl(WorldSys)[-]"
  RoadIncl(WorldSys)[-]___UNIQUE_1/1 -> __TDD__Tire.RoadIncl(WorldSys)[-]/1
  __TDD__Tire.RoadSlope(WorldSys)[-]/1 -> __TDO__Tire/15  "RoadSlope(WorldSys)[-]"
  RoadSlope(WorldSys)[-]___UNIQUE_1/1 -> __TDD__Tire.RoadSlope(WorldSys)[-]/1
  __TDD__Tire.ContactPointPos(WorldSys)[m]/1 -> __TDO__Tire/14  "ContactPointPos(WorldSys)[m]"
  ContactPointPos(WorldSys)[m]___UNIQUE_1/1 -> __TDD__Tire.ContactPointPos(WorldSys)[m]/1
  __TDD__Tire.RoadFrictionScalingCoeff[-]/1 -> __TDO__Tire/13  "RoadFrictionScalingCoeff[-]"
  RoadFrictionScalingCoeff[-]___UNIQUE_1/1 -> __TDD__Tire.RoadFrictionScalingCoeff[-]/1
  __TDD__Tire.RoadType[-]/1 -> __TDO__Tire/12  "RoadType[-]"
  RoadType[-]___UNIQUE_1/1 -> __TDD__Tire.RoadType[-]/1
  __TDD__Tire.RoadNormalVector(WorldSys)[-]/1 -> __TDO__Tire/11  "RoadNormalVector(WorldSys)[-]"
  RoadNormalVector(WorldSys)[-]___UNIQUE_1/1 -> __TDD__Tire.RoadNormalVector(WorldSys)[-]/1
  __TDD__Tire.LatUnitVector(WorldSys)[-]/1 -> __TDO__Tire/10  "LatUnitVector(WorldSys)[-]"
  LatUnitVector(WorldSys)[-]___UNIQUE_1/1 -> __TDD__Tire.LatUnitVector(WorldSys)[-]/1
  __TDD__Tire.LongUnitVector(WorldSys)[-]/1 -> __TDO__Tire/9  "LongUnitVector(WorldSys)[-]"
  LongUnitVector(WorldSys)[-]___UNIQUE_1/1 -> __TDD__Tire.LongUnitVector(WorldSys)[-]/1
  __TDD__Tire.LongFrcLeverArm_wrt_WheelRotAxis[m]/1 -> __TDO__Tire/8  "LongFrcLeverArm_wrt_WheelRotAxis[m]"
  LongFrcLeverArm_wrt_WheelRotAxis[m]___UNIQUE_1/1 -> __TDD__Tire.LongFrcLeverArm_wrt_WheelRotAxis[m]/1
  __TDD__Tire.BoreSpd(ContactSys)[rad/s]/1 -> __TDO__Tire/7  "BoreSpd(ContactSys)[rad/s]"
  BoreSpd(ContactSys)[rad/s]___UNIQUE_1/1 -> __TDD__Tire.BoreSpd(ContactSys)[rad/s]/1
  __TDD__Tire.LatSpd(ContactSys)[m/s]/1 -> __TDO__Tire/6  "LatSpd(ContactSys)[m/s]"
  LatSpd(ContactSys)[m/s]___UNIQUE_1/1 -> __TDD__Tire.LatSpd(ContactSys)[m/s]/1
  __TDD__Tire.LongSpd(ContactSys)[m/s]/1 -> __TDO__Tire/5  "LongSpd(ContactSys)[m/s]"
  LongSpd(ContactSys)[m/s]___UNIQUE_1/1 -> __TDD__Tire.LongSpd(ContactSys)[m/s]/1
  __TDD__Tire.TireDeflSpd[m/s]/1 -> __TDO__Tire/4  "TireDeflSpd[m/s]"
  TireDeflSpd[m/s]___UNIQUE_1/1 -> __TDD__Tire.TireDeflSpd[m/s]/1
  __TDD__Tire.TireDefl[m]/1 -> __TDO__Tire/3  "TireDefl[m]"
  TireDefl[m]___UNIQUE_1/1 -> __TDD__Tire.TireDefl[m]/1
  __TDD__Tire.CamberAng(ContactSys)[rad]/1 -> __TDO__Tire/2  "CamberAng(ContactSys)[rad]"
  CamberAng(ContactSys)[rad]___UNIQUE_1/1 -> __TDD__Tire.CamberAng(ContactSys)[rad]/1
  __TDD__Tire.ContactPointPos_wrt_WheelCenter(WorldSys)[m]/1 -> __TDO__Tire/1  "ContactPointPos_wrt_WheelCenter(WorldSys)[m]"
  ContactPointPos_wrt_WheelCenter(WorldSys)[m]___UNIQUE_1/1 -> __TDD__Tire.ContactPointPos_wrt_WheelCenter(WorldSys)[m]/1

== system SingleTrackCANoe/SimulationModel/Vehicle/WheelSystem/FrontRightWheelSystem/Tire/DynaComponentInfo ==

== system SingleTrackCANoe/SimulationModel/Vehicle/WheelSystem/FrontRightWheelSystem/Tire/InputFromCTRL ==
  fromCTRL : Inport
  TDBusSelector : BusSelector  OutputSignals=AddRoadElev[m],RoadFrictionScaling[0_2],AddLongRoadSlope[-],AddLatRoadSlope[-],LocalRoadSysSwitch[0;1]
  __TDD__AddLatRoadSlope[-] : Demux  Outputs=[1]
  __TDD__AddLongRoadSlope[-] : Demux  Outputs=[1]
  __TDD__AddRoadElev[m] : Demux  Outputs=[1]
  __TDD__LocalRoadSysSwitch[0;1] : Demux  Outputs=[1]
  __TDD__RoadFrictionScaling[0_2] : Demux  Outputs=[1]
  AddRoadElev[m]___UNIQUE_1 : Outport  Description=|  PortDimensions=[1]  VectorParamsAs1DForOutWhenUnconnected=off
      | <name>AddRoadElev[m]</name>
      | <comment></comment>
  RoadFrictionScaling[0_2]___UNIQUE_1 : Outport  Description=|  Port=2  PortDimensions=[1]  VectorParamsAs1DForOutWhenUnconnected=off
      | <name>RoadFrictionScaling[0_2]</name>
      | <comment></comment>
  AddLongRoadSlope[-]___UNIQUE_1 : Outport  Description=|  Port=3  PortDimensions=[1]  VectorParamsAs1DForOutWhenUnconnected=off
      | <name>AddLongRoadSlope[-]</name>
      | <comment></comment>
  AddLatRoadSlope[-]___UNIQUE_1 : Outport  Description=|  Port=4  PortDimensions=[1]  VectorParamsAs1DForOutWhenUnconnected=off
      | <name>AddLatRoadSlope[-]</name>
      | <comment></comment>
  LocalRoadSysSwitch[0;1]___UNIQUE_1 : Outport  Description=|  Port=5  PortDimensions=[1]  VectorParamsAs1DForOutWhenUnconnected=off
      | <name>LocalRoadSysSwitch[0;1]</name>
      | <comment></comment>
  wires:
  fromCTRL/1 -> TDBusSelector/1
  TDBusSelector/1 -> __TDD__AddRoadElev[m]/1  "<AddRoadElev[m]>"
  TDBusSelector/2 -> __TDD__RoadFrictionScaling[0_2]/1  "<RoadFrictionScaling[0_2]>"
  TDBusSelector/3 -> __TDD__AddLongRoadSlope[-]/1  "<AddLongRoadSlope[-]>"
  TDBusSelector/4 -> __TDD__AddLatRoadSlope[-]/1  "<AddLatRoadSlope[-]>"
  TDBusSelector/5 -> __TDD__LocalRoadSysSwitch[0;1]/1  "<LocalRoadSysSwitch[0;1]>"
  __TDD__AddRoadElev[m]/1 -> AddRoadElev[m]___UNIQUE_1/1  "AddRoadElev[m]"
  __TDD__RoadFrictionScaling[0_2]/1 -> RoadFrictionScaling[0_2]___UNIQUE_1/1  "RoadFrictionScaling[0_2]"
  __TDD__AddLongRoadSlope[-]/1 -> AddLongRoadSlope[-]___UNIQUE_1/1  "AddLongRoadSlope[-]"
  __TDD__AddLatRoadSlope[-]/1 -> AddLatRoadSlope[-]___UNIQUE_1/1  "AddLatRoadSlope[-]"
  __TDD__LocalRoadSysSwitch[0;1]/1 -> LocalRoadSysSwitch[0;1]___UNIQUE_1/1  "LocalRoadSysSwitch[0;1]"

== system SingleTrackCANoe/SimulationModel/Vehicle/WheelSystem/FrontRightWheelSystem/Tire/InputFromChassis ==
  fromChassis : Inport
  TDBusSelector : BusSelector  OutputSignals=VehicleBody.PosAxleSys(WorldSys),VehicleBody.RotMatrix(WorldSys)[-],WheelSystem.WheelRotAxis(VehSys)[-],WheelSystem.TirePos(AxleSys)[m],WheelSystem.TireVel_wrt_WorldSys(VehSys)[m/s],WheelSystem.WheelRotVel_wrt_WorldSys(VehSys)[rad/s],VehicleBody.Vel_wrt_WorldSys(VehSys)[m/s],WheelSystem.WheelRotMatrix(WorldSys)[-],WheelSystem.TireDefl[m]
  __TDD__PosAxleSys(WorldSys) : Demux  Outputs=1
  __TDD__RotMatrix(WorldSys)[-] : Demux  Outputs=[9]
  __TDD__TireDefl[m] : Demux  Outputs=[1]
  __TDD__TirePos(AxleSys)[m] : Demux  Outputs=1
  __TDD__TireVel_wrt_WorldSys(VehSys)[m/s] : Demux  Outputs=[3]
  __TDD__Vel_wrt_WorldSys(VehSys)[m/s] : Demux  Outputs=[3]
  __TDD__WheelRotAxis(VehSys)[-] : Demux  Outputs=[3]
  __TDD__WheelRotMatrix(WorldSys)[-] : Demux  Outputs=[9]
  __TDD__WheelRotVel_wrt_WorldSys(VehSys)[rad/s] : Demux  Outputs=[3]
  PosAxleSys(WorldSys)___UNIQUE_1 : Outport  Description=|  VectorParamsAs1DForOutWhenUnconnected=off
      | <name>VehicleBody.PosAxleSys(WorldSys)</name>
      | <comment></comment>
  RotMatrix(WorldSys)[-]___UNIQUE_1 : Outport  Description=|  Port=2  PortDimensions=[9]  VectorParamsAs1DForOutWhenUnconnected=off
      | <name>VehicleBody.RotMatrix(WorldSys)[-]</name>
      | <comment></comment>
  WheelRotAxis(VehSys)[-]___UNIQUE_1 : Outport  Description=|  Port=3  PortDimensions=[3]  VectorParamsAs1DForOutWhenUnconnected=off
      | <name>WheelSystem.WheelRotAxis(VehSys)[-]</name>
      | <comment></comment>
  TirePos(AxleSys)[m]___UNIQUE_1 : Outport  Description=|  Port=4  VectorParamsAs1DForOutWhenUnconnected=off
      | <name>WheelSystem.TirePos(AxleSys)[m]</name>
      | <comment></comment>
  TireVel_wrt_WorldSys(VehSys)[m/s]___UNIQUE_1 : Outport  Description=|  Port=5  PortDimensions=[3]  VectorParamsAs1DForOutWhenUnconnected=off
      | <name>WheelSystem.TireVel_wrt_WorldSys(VehSys)[m/s]</name>
      | <comment></comment>
  WheelRotVel_wrt_WorldSys(VehSys)[rad/s]___UNIQUE_1 : Outport  Description=|  Port=6  PortDimensions=[3]  VectorParamsAs1DForOutWhenUnconnected=off
      | <name>WheelSystem.WheelRotVel_wrt_WorldSys(VehSys)[rad/s]</name>
      | <comment></comment>
  Vel_wrt_WorldSys(VehSys)[m/s]___UNIQUE_1 : Outport  Description=|  Port=7  PortDimensions=[3]  VectorParamsAs1DForOutWhenUnconnected=off
      | <name>VehicleBody.Vel_wrt_WorldSys(VehSys)[m/s]</name>
      | <comment></comment>
  WheelRotMatrix(WorldSys)[-]___UNIQUE_1 : Outport  Description=|  Port=8  PortDimensions=[9]  VectorParamsAs1DForOutWhenUnconnected=off
      | <name>WheelSystem.WheelRotMatrix(WorldSys)[-]</name>
      | <comment></comment>
  TireDefl[m]___UNIQUE_1 : Outport  Description=|  Port=9  PortDimensions=[1]  VectorParamsAs1DForOutWhenUnconnected=off
      | <name>WheelSystem.TireDefl[m]</name>
      | <comment></comment>
  wires:
  fromChassis/1 -> TDBusSelector/1
  TDBusSelector/1 -> __TDD__PosAxleSys(WorldSys)/1  "<PosAxleSys(WorldSys)>"
  TDBusSelector/2 -> __TDD__RotMatrix(WorldSys)[-]/1  "<RotMatrix(WorldSys)[-]>"
  TDBusSelector/3 -> __TDD__WheelRotAxis(VehSys)[-]/1  "<WheelRotAxis(VehSys)[-]>"
  TDBusSelector/4 -> __TDD__TirePos(AxleSys)[m]/1  "<TirePos(AxleSys)[m]>"
  TDBusSelector/5 -> __TDD__TireVel_wrt_WorldSys(VehSys)[m/s]/1  "<TireVel_wrt_WorldSys(VehSys)[m/s]>"
  TDBusSelector/6 -> __TDD__WheelRotVel_wrt_WorldSys(VehSys)[rad/s]/1  "<WheelRotVel_wrt_WorldSys(VehSys)[rad/s]>"
  TDBusSelector/7 -> __TDD__Vel_wrt_WorldSys(VehSys)[m/s]/1  "<Vel_wrt_WorldSys(VehSys)[m/s]>"
  TDBusSelector/8 -> __TDD__WheelRotMatrix(WorldSys)[-]/1  "<WheelRotMatrix(WorldSys)[-]>"
  TDBusSelector/9 -> __TDD__TireDefl[m]/1  "<TireDefl[m]>"
  __TDD__PosAxleSys(WorldSys)/1 -> PosAxleSys(WorldSys)___UNIQUE_1/1  "PosAxleSys(WorldSys)"
  __TDD__RotMatrix(WorldSys)[-]/1 -> RotMatrix(WorldSys)[-]___UNIQUE_1/1  "RotMatrix(WorldSys)[-]"
  __TDD__WheelRotAxis(VehSys)[-]/1 -> WheelRotAxis(VehSys)[-]___UNIQUE_1/1  "WheelRotAxis(VehSys)[-]"
  __TDD__TirePos(AxleSys)[m]/1 -> TirePos(AxleSys)[m]___UNIQUE_1/1  "TirePos(AxleSys)[m]"
  __TDD__TireVel_wrt_WorldSys(VehSys)[m/s]/1 -> TireVel_wrt_WorldSys(VehSys)[m/s]___UNIQUE_1/1  "TireVel_wrt_WorldSys(VehSys)[m/s]"
  __TDD__WheelRotVel_wrt_WorldSys(VehSys)[rad/s]/1 -> WheelRotVel_wrt_WorldSys(VehSys)[rad/s]___UNIQUE_1/1  "WheelRotVel_wrt_WorldSys(VehSys)[rad/s]"
  __TDD__Vel_wrt_WorldSys(VehSys)[m/s]/1 -> Vel_wrt_WorldSys(VehSys)[m/s]___UNIQUE_1/1  "Vel_wrt_WorldSys(VehSys)[m/s]"
  __TDD__WheelRotMatrix(WorldSys)[-]/1 -> WheelRotMatrix(WorldSys)[-]___UNIQUE_1/1  "WheelRotMatrix(WorldSys)[-]"
  __TDD__TireDefl[m]/1 -> TireDefl[m]___UNIQUE_1/1  "TireDefl[m]"

== system SingleTrackCANoe/SimulationModel/Vehicle/WheelSystem/FrontRightWheelSystem/Tire/InputFromWheel ==
  fromWheel : Inport
  TDBusSelector : BusSelector  OutputSignals=RotSpd[rad/s],BlockingState[0;1]
  __TDD__BlockingState[0;1] : Demux  Outputs=[1]
  __TDD__RotSpd[rad/s] : Demux  Outputs=[1]
  RotSpd[rad/s]___UNIQUE_1 : Outport  Description=|  PortDimensions=[1]  VectorParamsAs1DForOutWhenUnconnected=off
      | <name>RotSpd[rad/s]</name>
      | <comment></comment>
  BlockingState[0;1]___UNIQUE_1 : Outport  Description=|  Port=2  PortDimensions=[1]  VectorParamsAs1DForOutWhenUnconnected=off
      | <name>BlockingState[0;1]</name>
      | <comment></comment>
  wires:
  fromWheel/1 -> TDBusSelector/1
  TDBusSelector/1 -> __TDD__RotSpd[rad/s]/1  "<RotSpd[rad/s]>"
  TDBusSelector/2 -> __TDD__BlockingState[0;1]/1  "<BlockingState[0;1]>"
  __TDD__RotSpd[rad/s]/1 -> RotSpd[rad/s]___UNIQUE_1/1  "RotSpd[rad/s]"
  __TDD__BlockingState[0;1]/1 -> BlockingState[0;1]___UNIQUE_1/1  "BlockingState[0;1]"
